simulink model "hollow"  (R2024a)
settings: Solver=ode45  StartTime=0  StopTime=500  FixedStep=0.01  MaxStep=0.01  RelTol=1e-3  EnableMultiTasking=on
values from neighbouring files (symbols this model uses):
  simu = simulationClass()    [wecSimInputFile.m]
undefined symbols (not defined in the file or in its folder): body, constraint, mooring, pto, ptoCoeffcient
libraries: WECSim_Lib_Body_Elements x4, WECSim_Lib_PTOs x3, WECSim_Lib_Constraints x1, WECSim_Lib_Frames x1, WECSim_Lib_Moorings x1
settings Model: Creator=mlawson  LastModifiedBy=rithikrn
settings SolverCC: ZeroCrossControl=DisableAll  AlgebraicLoopSolver=LineSearch  AutoInsertRateTranBlk=on
settings DataIOCC: SaveFormat=Array  SaveOutput=off  SaveTime=off  ReturnWorkspaceOutputs=off
settings OptimizationCC: LifeSpan=inf  SimCompilerOptimization=on
settings DebuggingCC: MergeDetectMultiDrivingBlocksExec=none  SolverPrmCheckMsg=warning  UnconnectedInputMsg=warning  UnconnectedOutputMsg=warning  UnconnectedLineMsg=warning  AllowSymbolicDim=off  StateNameClashWarn=warning  SFUnexpectedBacktrackingDiag=warning  SFNoUnconditionalDefaultTransitionDiag=warning  SFExecutionAtInitializationDiag=none  ArithmeticOperatorsInVariantConditions=warning
settings HardwareCC: ProdBitPerPointer=32  ProdBitPerSizeT=32  ProdBitPerPtrDiffT=32  ProdLargestAtomicFloat=None  ProdIntDivRoundTo=Undefined  ProdEndianess=Unspecified  ProdWordSize=32  ProdHWDeviceType=32-bit Generic
settings ModelReferenceCC: EnableRefExpFcnMdlSchedulingChecks=on  PropagateSignalLabelsOutOfModel=off
settings SFSimCC: SimUseLocalCustomCode=off  CustomCodeUndefinedFunction=UseInterfaceOnly
settings RTWCC: RTWUseLocalCustomCode=off  GPUComputeCapability=3.5
settings CodeAppCC: StateflowObjectComments=on
settings GRTTargetCC: TargetLangStandard=C89/C90 (ANSI)
settings ConfigComp: CovMetricSettings=dw  CovSaveCumulativeToWorkspaceVar=on  CovSaveSingleToWorkspaceVar=on  CovExternalEMLEnable=off  CovSFcnEnable=off
settings SimscapeCC: SimscapeNormalizeSystem=off
settings ConfigurationSet: Description=SimMechanics 2G
settings ExplorerConfigSet: InternalSimMechanicsExplorerSettings="<ExplorerConfiguration><canonicalview>default</canonicalview><TilePanel><TileInfo><Tiles Columns=\"1\" Count=\"1\" Rows=\"1\"><Column Left=\"2\" Weight=\"1\"/><Column Left=\"1335\"/><Row Top=\"2\" Weight=\"1\"/><Row Top=\"911\"/><Tile Height=\"1\" Width=\"1\" X=\"0\" Y=\"0\"/></Tiles></TileInfo><SceneInfo><SceneViewer><BGColor><R>0.60000002384185791</R><G>0.60000002384185791</G><B>0.60000002384185791</B></BGColor><Camera><Position><X>365.37645888990272</X><Y>-369.82486814446582</Y><Z>359.64809521743916</Z></Position><Center><X>-6.7351450971904585</X><Y>2.2867358426280204</Y><Z>-12.463508769654169</Z></Center><Up><X>-0.40824829046386307</X><Y>0.40824829046386307</Y><Z>0.81649658092772615</Z></Up><Left>-57.820127362122818</Left><Right>57.820127362122818</Right><Bottom>-38.308817187253304</Bottom><Top>38.308817187253304</Top></Camera></SceneViewer></SceneInfo></TilePanel></ExplorerConfiguration>"

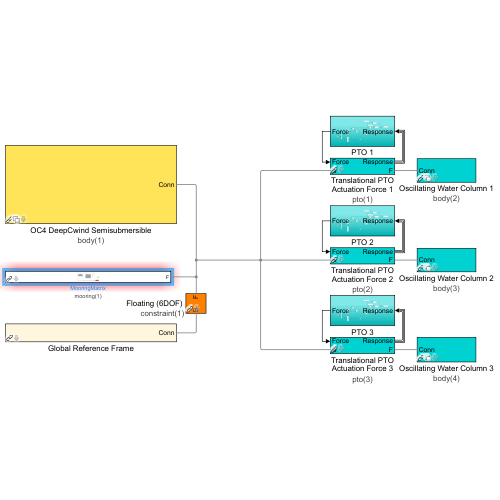
[thumbnail: Simulink's stored preview of the top-level diagram]
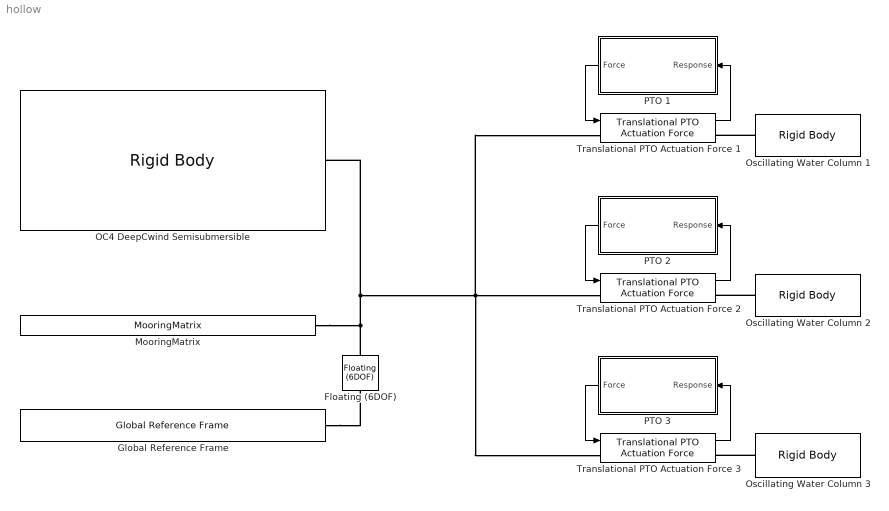
== system hollow ==
  Floating (6DOF) : WECSim_Lib_Constraints/Floating (6DOF)  constraint=constraint(1)
      settings: AttributesFormatString=%<constraint>
  Global Reference Frame : WECSim_Lib_Frames/Global Reference Frame  waves=waves  simu=simu
  MooringMatrix : WECSim_Lib_Moorings/MooringMatrix  mooring=mooring(1)  loc=0 0 0  preTension=[0 0 0 0 0 0]  stiffness={ '0', '0', '0', '0', '0', '0'; '0', '0', '0', '0', '0', '0'; '0', '0', '0', '0', '0', '0'; '0', '0', '0', '0', '0', '0'; '0', '0', '0', '0', '0', '0'; '0', '0', '0', '0', '0', '0' }  damping={ '0', '0', '0', '0', '0', '0'; '0', '0', '0', '0', '0', '0'; '0', '0', '0', '0', '0', '0'; '0', '0', '0', '0', '0', '0'; '0', '0', '0', '0', '0', '0'; '0', '0', '0', '0', '0', '0' }
      settings: AttributesFormatString=%<mooring>
  OC4 DeepCwind Semisubmersible : WECSim_Lib_Body_Elements/Rigid Body  body=body(1)
  Oscillating Water Column 1 : WECSim_Lib_Body_Elements/Rigid Body  body=body(2)
  Oscillating Water Column 2 : WECSim_Lib_Body_Elements/Rigid Body  body=body(3)
  Oscillating Water Column 3 : WECSim_Lib_Body_Elements/Rigid Body  body=body(4)
  PTO 1 : Subsystem
  PTO 2 : Subsystem
  PTO 3 : Subsystem
  Translational PTO Actuation Force 1 : WECSim_Lib_PTOs/Translational PTO Actuation Force  pto=pto(1)
      settings: AttributesFormatString=%<pto>
  Translational PTO Actuation Force 2 : WECSim_Lib_PTOs/Translational PTO Actuation Force  pto=pto(2)
      settings: AttributesFormatString=%<pto>
  Translational PTO Actuation Force 3 : WECSim_Lib_PTOs/Translational PTO Actuation Force  pto=pto(3)
      settings: AttributesFormatString=%<pto>
  wires:
  Translational PTO Actuation Force 1/1 -> PTO 1/1(Response)
  PTO 1/1(Force) -> Translational PTO Actuation Force 1/1
  PTO 2/1(Force) -> Translational PTO Actuation Force 2/1
  Translational PTO Actuation Force 2/1 -> PTO 2/1(Response)
  PTO 3/1(Force) -> Translational PTO Actuation Force 3/1
  Translational PTO Actuation Force 3/1 -> PTO 3/1(Response)
  connections:
  Global Reference Frame/RConn1 -- Floating (6DOF)/LConn1
  Floating (6DOF)/RConn1 -- MooringMatrix/LConn1 -- OC4 DeepCwind Semisubmersible/RConn1 -- Translational PTO Actuation Force 2/LConn1 -- Translational PTO Actuation Force 1/LConn1 -- Translational PTO Actuation Force 3/LConn1
  Oscillating Water Column 3/RConn1 -- Translational PTO Actuation Force 3/RConn1
  Oscillating Water Column 2/RConn1 -- Translational PTO Actuation Force 2/RConn1
  Oscillating Water Column 1/RConn1 -- Translational PTO Actuation Force 1/RConn1

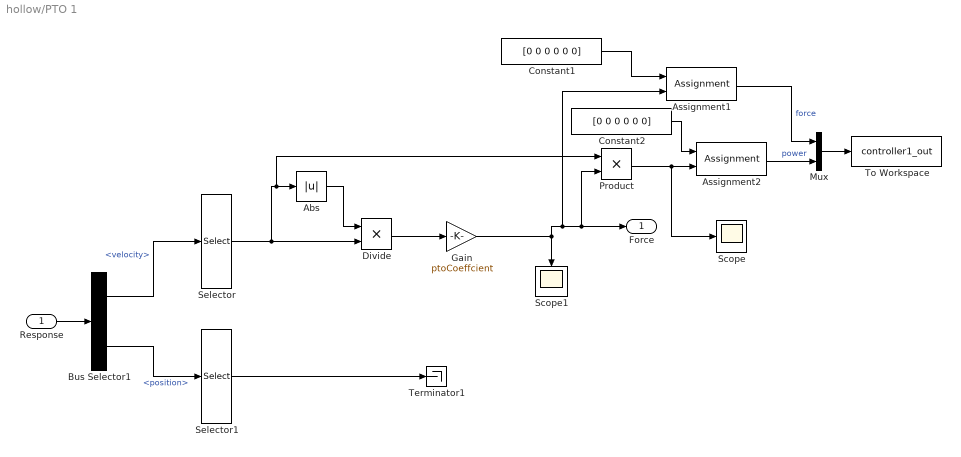
== system hollow/PTO 1 ==
  Response : Inport
  Abs : Abs  SaturateOnIntegerOverflow=off
  Assignment1 : Assignment  IndexOptions=Index vector (dialog)  Indices=3  OutputSizes=1
  Assignment2 : Assignment  IndexOptions=Index vector (dialog)  Indices=3  OutputSizes=1
  Bus Selector1 : BusSelector  OutputSignals=velocity,position
  Constant1 : Constant  Value=[0 0 0 0 0 0]
  Constant2 : Constant  Value=[0 0 0 0 0 0]
  Divide : Product  Inputs=**
  Gain : Gain  Gain=ptoCoeffcient
  Mux : Mux  Inputs=2
  Product : Product
  Scope : Scope
  Scope1 : Scope
  Selector : Selector  InputPortWidth=6  IndexOptions=Index vector (dialog)  Indices=3  OutputSizes=1
  Selector1 : Selector  InputPortWidth=6  IndexOptions=Index vector (dialog)  Indices=3  OutputSizes=1
  Terminator1 : Terminator
  To Workspace : ToWorkspace  VariableName=controller1_out  SaveFormat=Structure With Time  SampleTime=simu.dtOut
  Force : Outport
  wires:
  Bus Selector1/1 -> Selector/1  "<velocity>"
  Constant2/1 -> Assignment2/1
  Assignment1/1 -> Mux/1  "force"
  Assignment2/1 -> Mux/2  "power"
  Constant1/1 -> Assignment1/1
  Mux/1 -> To Workspace/1
  Bus Selector1/2 -> Selector1/1  "<position>"
  Response/1 -> Bus Selector1/1
  Selector1/1 -> Terminator1/1
  Gain/1 -> Assignment1/2, Force/1, Product/2, Scope1/1
  Selector/1 -> Product/1, Abs/1, Divide/2
  Abs/1 -> Divide/1
  Divide/1 -> Gain/1
  Product/1 -> Scope/1, Assignment2/2

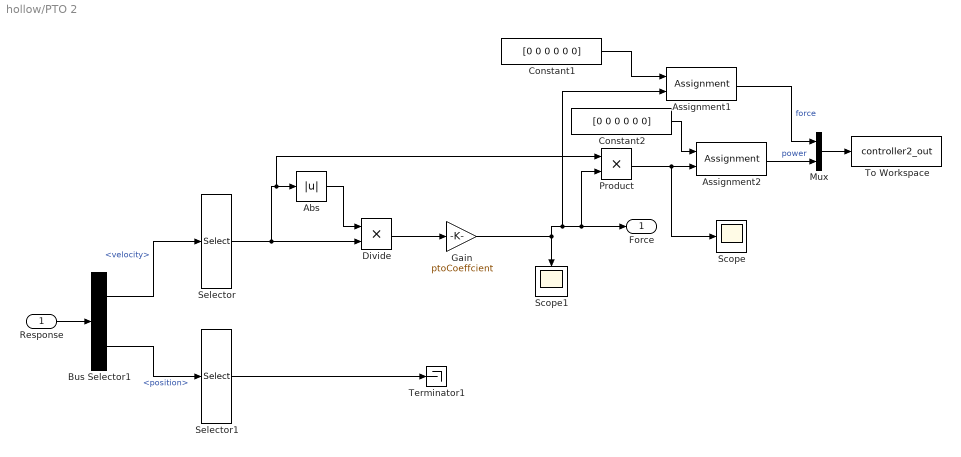
== system hollow/PTO 2 ==
  Response : Inport
  Abs : Abs  SaturateOnIntegerOverflow=off
  Assignment1 : Assignment  IndexOptions=Index vector (dialog)  Indices=3  OutputSizes=1
  Assignment2 : Assignment  IndexOptions=Index vector (dialog)  Indices=3  OutputSizes=1
  Bus Selector1 : BusSelector  OutputSignals=velocity,position
  Constant1 : Constant  Value=[0 0 0 0 0 0]
  Constant2 : Constant  Value=[0 0 0 0 0 0]
  Divide : Product  Inputs=**
  Gain : Gain  Gain=ptoCoeffcient
  Mux : Mux  Inputs=2
  Product : Product
  Scope : Scope
  Scope1 : Scope
  Selector : Selector  InputPortWidth=6  IndexOptions=Index vector (dialog)  Indices=3  OutputSizes=1
  Selector1 : Selector  InputPortWidth=6  IndexOptions=Index vector (dialog)  Indices=3  OutputSizes=1
  Terminator1 : Terminator
  To Workspace : ToWorkspace  VariableName=controller2_out  SaveFormat=Structure With Time  SampleTime=simu.dtOut
  Force : Outport
  wires:
  Bus Selector1/1 -> Selector/1  "<velocity>"
  Constant2/1 -> Assignment2/1
  Assignment1/1 -> Mux/1  "force"
  Assignment2/1 -> Mux/2  "power"
  Constant1/1 -> Assignment1/1
  Mux/1 -> To Workspace/1
  Bus Selector1/2 -> Selector1/1  "<position>"
  Response/1 -> Bus Selector1/1
  Selector1/1 -> Terminator1/1
  Gain/1 -> Assignment1/2, Force/1, Product/2, Scope1/1
  Selector/1 -> Product/1, Abs/1, Divide/2
  Abs/1 -> Divide/1
  Divide/1 -> Gain/1
  Product/1 -> Scope/1, Assignment2/2

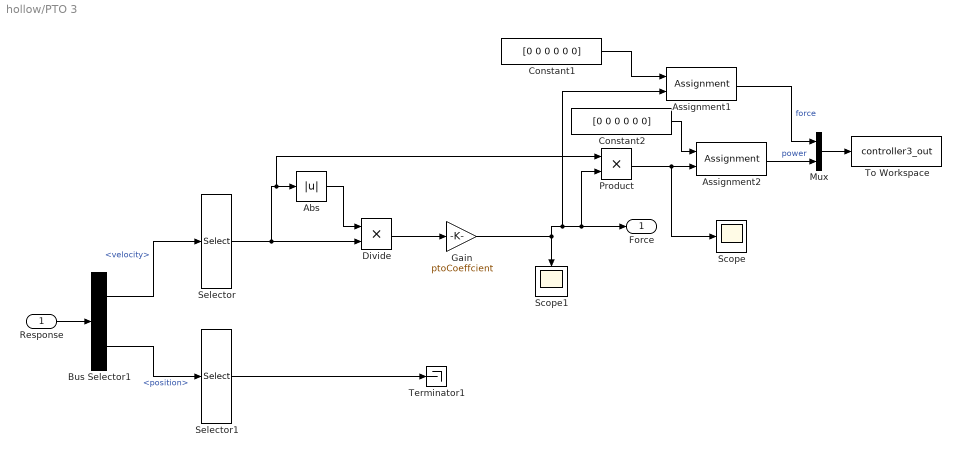
== system hollow/PTO 3 ==
  Response : Inport
  Abs : Abs  SaturateOnIntegerOverflow=off
  Assignment1 : Assignment  IndexOptions=Index vector (dialog)  Indices=3  OutputSizes=1
  Assignment2 : Assignment  IndexOptions=Index vector (dialog)  Indices=3  OutputSizes=1
  Bus Selector1 : BusSelector  OutputSignals=velocity,position
  Constant1 : Constant  Value=[0 0 0 0 0 0]
  Constant2 : Constant  Value=[0 0 0 0 0 0]
  Divide : Product  Inputs=**
  Gain : Gain  Gain=ptoCoeffcient
  Mux : Mux  Inputs=2
  Product : Product
  Scope : Scope
  Scope1 : Scope
  Selector : Selector  InputPortWidth=6  IndexOptions=Index vector (dialog)  Indices=3  OutputSizes=1
  Selector1 : Selector  InputPortWidth=6  IndexOptions=Index vector (dialog)  Indices=3  OutputSizes=1
  Terminator1 : Terminator
  To Workspace : ToWorkspace  VariableName=controller3_out  SaveFormat=Structure With Time  SampleTime=simu.dtOut
  Force : Outport
  wires:
  Bus Selector1/1 -> Selector/1  "<velocity>"
  Constant2/1 -> Assignment2/1
  Assignment1/1 -> Mux/1  "force"
  Assignment2/1 -> Mux/2  "power"
  Constant1/1 -> Assignment1/1
  Mux/1 -> To Workspace/1
  Bus Selector1/2 -> Selector1/1  "<position>"
  Response/1 -> Bus Selector1/1
  Selector1/1 -> Terminator1/1
  Gain/1 -> Assignment1/2, Force/1, Product/2, Scope1/1
  Selector/1 -> Product/1, Abs/1, Divide/2
  Abs/1 -> Divide/1
  Divide/1 -> Gain/1
  Product/1 -> Scope/1, Assignment2/2
